simulink model "mrSimulator"  (R2014a)
settings: Solver=ode45  StartTime=0.0  StopTime=60  RelTol=1e-3
InitFcn:
  | params
undefined symbols (not defined in the file or in its folder): mrAttitudeController, mrDrawAircraft, mrPositionController, P
libraries: simulink x8
settings Model: Creator=beard  LastModifiedBy=james
settings DataIOCC: SignalLoggingSaveFormat=ModelDataLogs
settings OptimizationCC: ExpressionDepthLimit=2147483647  InitFltsAndDblsToZero=on
settings DebuggingCC: UnderspecifiedInitializationDetection=Classic  MultiTaskDSMMsg=warning  MultiTaskCondExecSysMsg=none  FcnCallInpInsideContextMsg=UseLocalSettings  StateNameClashWarn=warning
settings SFSimCC: SimParseCustomCode=off
settings RTWCC: IncludeERTFirstTime=on
settings GRTTargetCC: CombineOutputUpdateFcns=off  GRTInterface=on

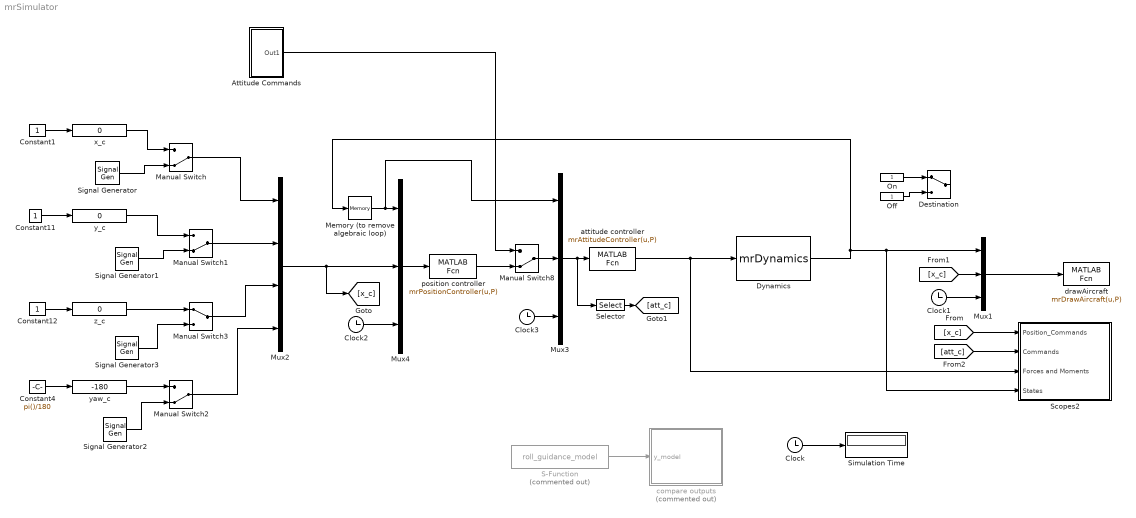
== system mrSimulator ==
  Attitude Commands : Subsystem
  Clock{,1..3} (4 alike) : Clock
  Constant1 : Constant
  Constant11 : Constant
  Constant12 : Constant
  Constant4 : Constant  Value=pi()/180
  Destination : ManualSwitch
  Dynamics : S-Function  FunctionName=mrDynamics  Parameters=P  EnableBusSupport=off
  Manual Switch{,1..2,8} (4 alike) : ManualSwitch  CurrentSetting=0
  Manual Switch3 : ManualSwitch
  Memory (to remove algebraic loop) : Memory
  Mux1 : Mux  Inputs=3
  Mux2 : Mux
  Mux3 : Mux  Inputs=3
  Mux4 : Mux  Inputs=3
  "Off " : Constant
  On : Constant
  S-Function : S-Function  Commented=on  FunctionName=roll_guidance_model  Parameters=P  EnableBusSupport=off
  Scopes2 : Subsystem
  Selector : Selector  Indices=[14 13 15 16]
  Signal Generator : SignalGenerator  WaveForm=square  Amplitude=25  Frequency=.05
  Signal Generator1 : SignalGenerator  WaveForm=square  Amplitude=15  Frequency=.0333
  Signal Generator2 : SignalGenerator  WaveForm=square  Amplitude=90*pi()/180  Frequency=.02
  Signal Generator3 : SignalGenerator  WaveForm=square  Amplitude=15  Frequency=.04
  Simulation Time : Display
  attitude controller : MATLABFcn  MATLABFcn=mrAttitudeController(u,P)  SampleTime=P.Ts
  compare outputs : Subsystem  Commented=on
  drawAircraft : MATLABFcn  MATLABFcn=mrDrawAircraft(u,P)  OutputDimensions=0  SampleTime=0.1
  position controller : MATLABFcn  MATLABFcn=mrPositionController(u,P)  OutputDimensions=4  SampleTime=P.Ts
  x_c : simulink/Math Operations/Slider Gain  low=-25  gain=0  high=25
  y_c : simulink/Math Operations/Slider Gain  low=-5  gain=0  high=5
  yaw_c : simulink/Math Operations/Slider Gain  low=-180  gain=-180  high=180
  z_c : simulink/Math Operations/Slider Gain  low=-5  gain=0  high=5
  wires:
  Clock/1 -> Simulation Time/1
  Constant1/1 -> x_c/1
  Constant11/1 -> y_c/1
  Constant12/1 -> z_c/1
  S-Function/1 -> compare outputs/1(y_model)
  Constant4/1 -> yaw_c/1
  Mux1/1 -> drawAircraft/1
  attitude controller/1 -> Dynamics/1, Scopes2/3(Forces and Moments)
  Memory (to remove algebraic loop)/1 -> Mux3/1, Mux4/1
  Clock2/1 -> Mux4/3
  Mux3/1 -> Selector/1, attitude controller/1
  Clock1/1 -> Mux1/3
  Clock3/1 -> Mux3/3
  Mux2/1 -> [x_c], Mux4/2
  Dynamics/1 -> Memory (to remove algebraic loop)/1, Mux1/1, Scopes2/4(States)
  [x_c] -> Scopes2/1(Position_Commands)
  [x_c] -> Mux1/2
  [att_c] -> Scopes2/2(Commands)
  Selector/1 -> [att_c]
  Signal Generator/1 -> Manual Switch/2
  x_c/1 -> Manual Switch/1
  Signal Generator1/1 -> Manual Switch1/2
  y_c/1 -> Manual Switch1/1
  Manual Switch1/1 -> Mux2/2
  Manual Switch/1 -> Mux2/1
  Manual Switch2/1 -> Mux2/4
  Manual Switch3/1 -> Mux2/3
  z_c/1 -> Manual Switch3/1
  Signal Generator3/1 -> Manual Switch3/2
  yaw_c/1 -> Manual Switch2/1
  Signal Generator2/1 -> Manual Switch2/2
  Mux4/1 -> position controller/1
  position controller/1 -> Manual Switch8/2
  Manual Switch8/1 -> Mux3/2
  On/1 -> Destination/1
  "Off "/1 -> Destination/2
  Attitude Commands/1(Out1) -> Manual Switch8/1

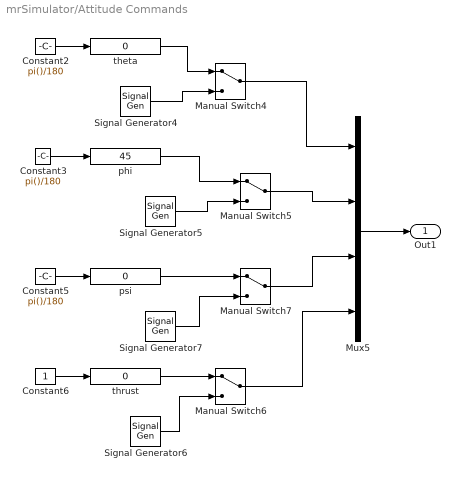
== system mrSimulator/Attitude Commands ==
  Constant2 : Constant  Value=pi()/180
  Constant3 : Constant  Value=pi()/180
  Constant5 : Constant  Value=pi()/180
  Constant6 : Constant
  Manual Switch{4..7} (4 alike) : ManualSwitch
  Mux5 : Mux
  Signal Generator4 : SignalGenerator  WaveForm=square  Amplitude=5  Frequency=.02
  Signal Generator5 : SignalGenerator  WaveForm=square  Amplitude=5  Frequency=.02
  Signal Generator6 : SignalGenerator  Amplitude=90  Frequency=.02
  Signal Generator7 : SignalGenerator  Amplitude=5  Frequency=.02
  phi : simulink/Math Operations/Slider Gain  low=-45  gain=45  high=45
  psi : simulink/Math Operations/Slider Gain  low=-5  gain=0  high=5
  theta : simulink/Math Operations/Slider Gain  low=-45  gain=0  high=45
  thrust : simulink/Math Operations/Slider Gain  low=0  gain=0  high=1
  Out1 : Outport
  wires:
  Constant2/1 -> theta/1
  Constant3/1 -> phi/1
  Constant5/1 -> psi/1
  Constant6/1 -> thrust/1
  Signal Generator4/1 -> Manual Switch4/2
  theta/1 -> Manual Switch4/1
  Signal Generator5/1 -> Manual Switch5/2
  phi/1 -> Manual Switch5/1
  Manual Switch5/1 -> Mux5/2
  Manual Switch4/1 -> Mux5/1
  Manual Switch6/1 -> Mux5/4
  Manual Switch7/1 -> Mux5/3
  psi/1 -> Manual Switch7/1
  Signal Generator7/1 -> Manual Switch7/2
  thrust/1 -> Manual Switch6/1
  Signal Generator6/1 -> Manual Switch6/2
  Mux5/1 -> Out1/1

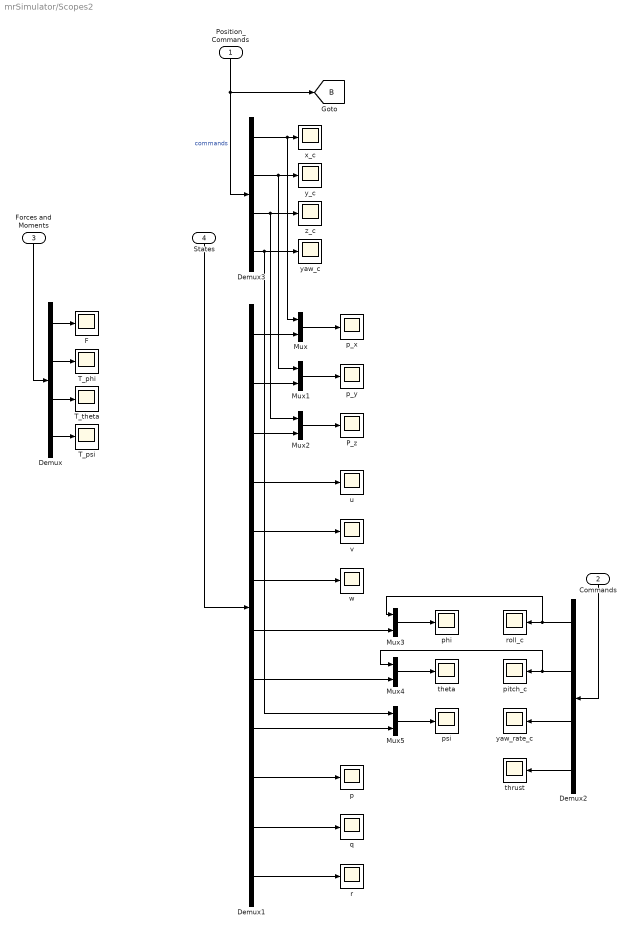
== system mrSimulator/Scopes2 ==
  Position_Commands : Inport
  Commands : Inport  Port=2
  Forces and Moments : Inport  Port=3
  States : Inport  Port=4
  Demux : Demux
  Demux1 : Demux  Outputs=12
  Demux2 : Demux
  Demux3 : Demux
  F : Scope
      settings: YMin=22.5  YMax=75
  Mux{,1..5} (6 alike) : Mux  Inputs=2
  P_z : Scope
      settings: TimeRange=60  YMin=0  YMax=3  SaveName=ScopeData6
  T_phi : Scope
  T_psi : Scope
      settings: SaveName=ScopeData3
  T_theta : Scope
      settings: SaveName=ScopeData2
  p : Scope
      settings: SaveName=ScopeData10
  p_x : Scope
      settings: YMin=-35  YMax=55  SaveName=ScopeData4
  p_y : Scope
      settings: TimeRange=60  YMin=-2.5  YMax=15  SaveName=ScopeData5
  phi : Scope
      settings: TimeRange=10  YMin=-1.75  YMax=1.75  SaveName=ScopeData13
  pitch_c : Scope
      settings: SaveName=ScopeData17
  psi : Scope
      settings: YMin=-1.75  YMax=1.75  SaveName=ScopeData15
  q : Scope
      settings: YMin=-0.175  YMax=0.2  SaveName=ScopeData11
  r : Scope
      settings: SaveName=ScopeData12
  roll_c : Scope
      settings: SaveName=ScopeData16
  theta : Scope
      settings: YMin=-1.4  YMax=0.6  SaveName=ScopeData14
  thrust : Scope
      settings: SaveName=ScopeData18
  u : Scope
      settings: SaveName=ScopeData7
  v : Scope
      settings: SaveName=ScopeData8
  w : Scope
      settings: SaveName=ScopeData9
  x_c : Scope
      settings: SaveName=ScopeData21
  y_c : Scope
      settings: SaveName=ScopeData20
  yaw_c : Scope
      settings: SaveName=ScopeData22
  yaw_rate_c : Scope
      settings: SaveName=ScopeData19
  z_c : Scope
      settings: SaveName=ScopeData23
  tag scope: B=global
  wires:
  States/1 -> Demux1/1
  Commands/1 -> Demux2/1
  Forces and Moments/1 -> Demux/1
  Demux/1 -> F/1
  Demux/4 -> T_psi/1
  Demux/2 -> T_phi/1
  Demux/3 -> T_theta/1
  Demux2/4 -> thrust/1
  Demux2/2 -> Mux4/1, pitch_c/1
  Demux2/3 -> yaw_rate_c/1
  Demux3/1 -> Mux/1, x_c/1
  Demux3/4 -> Mux5/1, yaw_c/1
  Demux3/2 -> Mux1/1, y_c/1
  Demux3/3 -> Mux2/1, z_c/1
  Mux/1 -> p_x/1
  Demux1/1 -> Mux/2
  Demux1/2 -> Mux1/2
  Demux1/3 -> Mux2/2
  Mux1/1 -> p_y/1
  Mux2/1 -> P_z/1
  Mux3/1 -> phi/1
  Mux4/1 -> theta/1
  Mux5/1 -> psi/1
  Demux1/4 -> u/1
  Demux1/5 -> v/1
  Demux1/6 -> w/1
  Demux1/10 -> p/1
  Demux1/11 -> q/1
  Demux1/12 -> r/1
  Demux1/9 -> Mux5/2
  Demux1/8 -> Mux4/2
  Demux1/7 -> Mux3/2
  Demux2/1 -> Mux3/1, roll_c/1
  Position_Commands/1 -> Demux3/1, [B]  "commands"

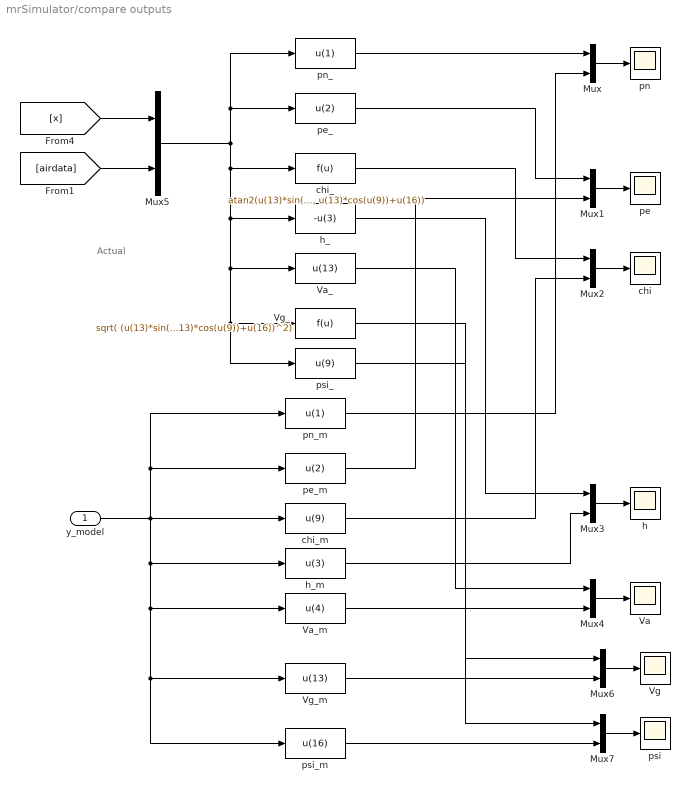
== system mrSimulator/compare outputs ==
  note: Actual
  y_model : Inport
  Mux{,1..7} (8 alike) : Mux  Inputs=2
  Va : Scope
      settings: TimeRange=40  YMin=29  YMax=42  SaveName=ScopeData4
  Va_ : Fcn  Expr=u(13)
  Va_m : Fcn  Expr=u(4)
  Vg : Scope
      settings: TimeRange=40  YMin=35  YMax=45  SaveName=ScopeData5
  Vg_ : Fcn  Expr=sqrt( (u(13)*sin(u(9))+u(17))^2+(u(13)*cos(u(9))+u(16))^2)
  Vg_m : Fcn  Expr=u(13)
  chi : Scope
      settings: TimeRange=40  YMin=-0.1  YMax=1.7  SaveName=ScopeData2
  chi_ : Fcn  Expr=atan2(u(13)*sin(u(9))+u(17), u(13)*cos(u(9))+u(16))
  chi_m : Fcn  Expr=u(9)
  h : Scope
      settings: TimeRange=115.3997603833866  YMin=0  YMax=110  SaveName=ScopeData3
  h_ : Fcn  Expr=-u(3)
  h_m : Fcn  Expr=u(3)
  pe : Scope
      settings: TimeRange=40  YMin=-100  YMax=250
  pe_ : Fcn  Expr=u(2)
  pe_m : Fcn  Expr=u(2)
  pn : Scope
      settings: TimeRange=40  YMin=-150  YMax=500
  pn_ : Fcn  Expr=u(1)
  pn_m : Fcn  Expr=u(1)
  psi : Scope
      settings: TimeRange=40  YMin=-0.25  YMax=1.75  SaveName=ScopeData6
  psi_ : Fcn  Expr=u(9)
  psi_m : Fcn  Expr=u(16)
  wires:
  pn_m/1 -> Mux/2
  chi_m/1 -> Mux2/2
  h_m/1 -> Mux3/2
  pe_m/1 -> Mux1/2
  Mux4/1 -> Va/1
  Mux3/1 -> h/1
  Mux2/1 -> chi/1
  Mux1/1 -> pe/1
  Mux/1 -> pn/1
  y_model/1 -> pn_m/1, pe_m/1, chi_m/1, h_m/1, Va_m/1, Vg_m/1, psi_m/1
  [x] -> Mux5/1
  [airdata] -> Mux5/2
  Mux5/1 -> pn_/1, pe_/1, h_/1, Va_/1, Vg_/1, psi_/1, chi_/1
  pn_/1 -> Mux/1
  pe_/1 -> Mux1/1
  Va_/1 -> Mux4/1
  h_/1 -> Mux3/1
  chi_/1 -> Mux2/1
  Vg_m/1 -> Mux6/2
  Mux6/1 -> Vg/1
  Vg_/1 -> Mux6/1
  psi_m/1 -> Mux7/2
  Mux7/1 -> psi/1
  psi_/1 -> Mux7/1
  Va_m/1 -> Mux4/2
